simulink model "radar_pipeline"  (R2025b)
settings: Solver=VariableStepAuto  StartTime=0.0  StopTime=0  RelTol=1e-3
libraries: dspxfrm3 x1, dspsigops x1
settings Model: Creator=T1983  LastModifiedBy=T1983
settings OptimizationCC: DefaultParameterBehavior=Inlined  EnhancedBackFolding=on  PassReuseOutputArgsAs=Individual arguments  ZeroExternalMemoryAtStartup=off  ZeroInternalMemoryAtStartup=off  OptimizeBlockOrder=speed  DifferentSizesBufferReuse=on  OptimizationCustomize=off  EfficientTunableParamExpr=on
settings DebuggingCC: ParameterTunabilityLossMsg=error
settings SFSimCC: SimCustomHeaderCode="#include \"doppler_processing.h\""  SimUserSources=../embedded_c/src/doppler_processing.c  SimUserIncludeDirs=../embedded_c/include  MATLABDynamicMemAlloc=off
settings RTWCC: SystemTargetFile=ert.tlc  TemplateMakefile=ert_default_tmf  Toolchain=MinGW64 | gmake (64-bit Windows)  Description=Embedded Coder
settings CodeAppCC: ForceParamTrailComments=on  IgnoreCustomStorageClasses=off  OperatorAnnotations=on  SimulinkDataObjDesc=on  SFDataObjDesc=on  InsertBlockDesc=on
settings ERTTargetCC: ERTCustomFileTemplate=example_file_process.tlc  TargetLangStandard=C99 (ISO)  GenerateSampleERTMain=on

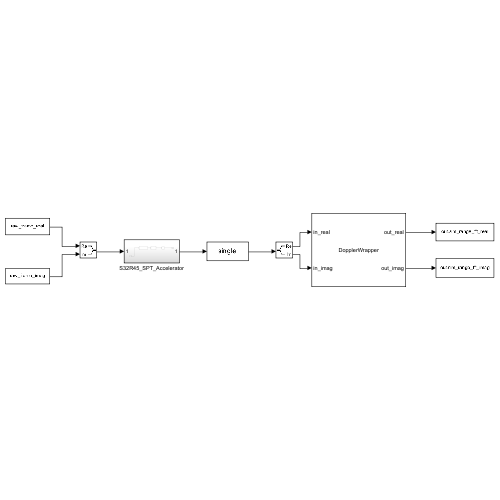
[thumbnail: Simulink's stored preview of the top-level diagram]
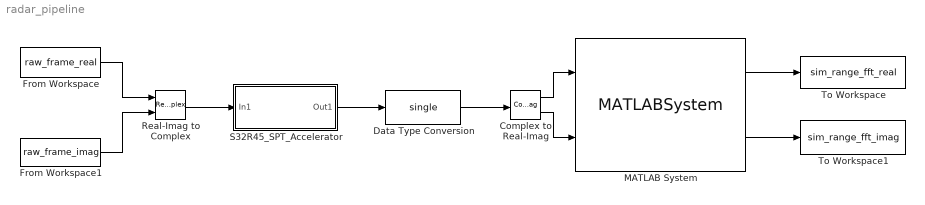
== system radar_pipeline ==
  Complex to Real-Imag : ComplexToRealImag
  Data Type Conversion : DataTypeConversion  OutDataTypeStr=single  SaturateOnIntegerOverflow=off  RndMeth=Floor
  From Workspace : FromWorkspace  VariableName=raw_frame_real
  From Workspace1 : FromWorkspace  VariableName=raw_frame_imag
  MATLAB System : MATLABSystem  System=DopplerWrapper  SimulateUsing=Code generation
      mask Type: DopplerWrapper
  Real-Imag to Complex : RealImagToComplex
  S32R45_SPT_Accelerator : Subsystem
  To Workspace : ToWorkspace  VariableName=sim_range_fft_real  SaveFormat=Timeseries  SampleTime=-1
  To Workspace1 : ToWorkspace  VariableName=sim_range_fft_imag  SaveFormat=Timeseries  SampleTime=-1
  wires:
  From Workspace/1 -> Real-Imag to Complex/1
  From Workspace1/1 -> Real-Imag to Complex/2
  Real-Imag to Complex/1 -> S32R45_SPT_Accelerator/1(In1)
  S32R45_SPT_Accelerator/1(Out1) -> Data Type Conversion/1
  Data Type Conversion/1 -> Complex to Real-Imag/1
  MATLAB System/1 -> To Workspace/1
  Complex to Real-Imag/1 -> MATLAB System/1
  Complex to Real-Imag/2 -> MATLAB System/2
  MATLAB System/2 -> To Workspace1/1

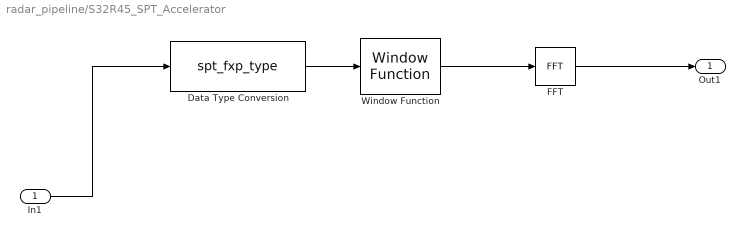
== system radar_pipeline/S32R45_SPT_Accelerator ==
  In1 : Inport
  Data Type Conversion : DataTypeConversion  OutDataTypeStr=spt_fxp_type  SaturateOnIntegerOverflow=off  RndMeth=Floor
  FFT : dspxfrm3/FFT  FFTImplementation=Auto  CompMethod=Table lookup  TableOpt=NEW  TableOptActive=Speed  BitRevOrder=off  Normalize=off  InheritFFTLength=on  FFTLength=64  WrapInput=on  roundingMode=Ceiling  overflowMode=on  firstCoeffDataTypeStr=Inherit: Same word length as input  firstCoeffLastDataTypeStr=Inherit: Same word length as input  outputMin=[]  outputMax=[]
      settings: LockScale=on
  Window Function : dspsigops/Window Function  winmode=Apply window to input  wintype=Hann  sampmode=Continuous  samptime=1  N=64  Rs=50  beta=10  winsamp=Periodic  UserWindow=hamming  OptParams=off  UserParams={'symmetric'}  dataType=double  isSigned=on  wordLen=16  udDataType=sfix(16)  fracBitsMode=Best precision  numFracBits=15  roundingMode=Floor  overflowMode=off  numSidelobes=4  sidelobeLevel=-30
  Out1 : Outport
  wires:
  In1/1 -> Data Type Conversion/1
  Data Type Conversion/1 -> Window Function/1
  Window Function/1 -> FFT/1
  FFT/1 -> Out1/1
